simulink model "hisf_0001_State_Machine_Type"  (R2018b)
settings: Solver=VariableStepAuto  StartTime=0.0  StopTime=10.0  RelTol=1e-3
settings Model: Creator=amyyang  LastModifiedBy=amyyang

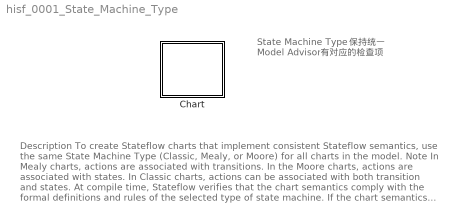
== system hisf_0001_State_Machine_Type ==
  note: State Machine Type 保持统一
      | Model Advisor有对应的检查项
  note: Description
      | To create Stateflow charts that implement consistent Stateflow semantics, use the
      | same State Machine Type (Classic, Mealy, or Moore) for all charts in the model.
      |
      | Note
      | In Mealy charts, actions are associated with transitions. In the Moore charts, actions
      | are associated with states. In Classic charts, actions can be associated with both
      | transition and states.
      | At compile time, Stateflow verifies that the chart semantics comply with the formal
      | definitions and rules of the selected type of state machine. If the chart semantics are
      | not in compliance, the software provides a diagnostic message.
      |
      | Rationale
      | Promote a clear modeling style.
  Chart : Stateflow chart  TreatAsAtomicUnit=on

== stateflow chart hisf_0001_State_Machine_Type/Chart ==
